simulink model "Simulinkrakata_lusail"  (R2024b)
settings: Solver=VariableStepAuto  StartTime=0.0  StopTime=700  RelTol=1e-3  AbsTol=1e-3
undefined symbols (not defined in the file or in its folder): coast_lookahead, lower_bound, throttle_slew, throttle_val, track_curvature, track_dist, track_slope, upper_bound
libraries: fl_lib x9, nesl_utility x9, sdl_lib x7, simulink x1, ee_lib x1
settings Model: Creator=ACER  LastModifiedBy=ACER
settings SolverCC: AutoScaleAbsTol=off  AlgebraicLoopSolver=TrustRegion  MaxZcPerStep=1
settings DebuggingCC: UnconnectedInputMsg=warning  UnconnectedOutputMsg=warning  UnconnectedLineMsg=warning  SymbolicDimsDataTypeCodeGenerationDiagnostic=none
settings ModelReferenceCC: EnableRefExpFcnMdlSchedulingChecks=on
settings SFSimCC: CustomCodeUndefinedFunction=UseInterfaceOnly
settings RTWCC: GPUComputeCapability=3.5  DLArmComputeVersion=19.05
settings SimscapeCC: SimscapeLogType=all  SimscapeLogSimulationStatistics=on  SimscapeLogDataHistory=10000

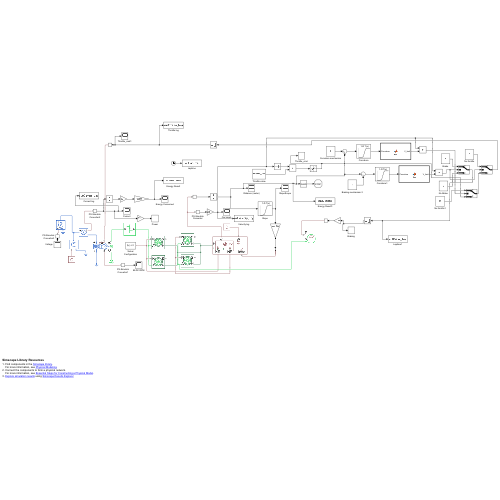
[thumbnail: Simulink's stored preview of the top-level diagram]
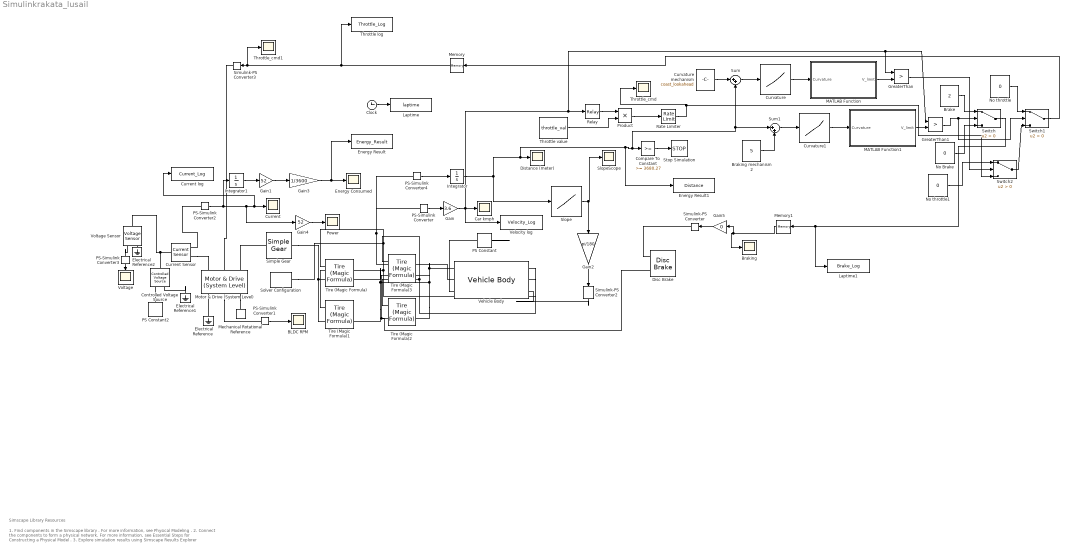
== system Simulinkrakata_lusail ==
  note: 1. Find components in the Simscape library .
      | For more information, see Physical Modeling .
      | 2. Connect the components to form a physical network.
      | For more information, see Essential Steps for Constructing a Physical Model .
      | 3. Explore simulation results using Simscape Results Explorer
  note: Simscape Library Resources
  BLDC RPM : Scope
  Brake : Constant  Value=2
  Braking : Scope
  Braking mechanism 2 : Constant  Value=5
  Car kmph : Scope
  Clock : Clock
  Compare To Constant : simulink/Logic and Bit Operations/Compare To Constant  relop=>=  const=3680.27  OutDataTypeStr=boolean
  Controlled Voltage Source : fl_lib/Electrical/Electrical Sources/Controlled Voltage Source
  Current : Scope
  Current Sensor : fl_lib/Electrical/Electrical Sensors/Current Sensor
  Current log : ToWorkspace  VariableName=Current_Log  SaveFormat=Timeseries  SampleTime=-1
  Curvature : Lookup_n-D  NumberOfTableDimensions=1  BreakpointsForDimension1=track_dist  Table=track_curvature  InternalRulePriority=Speed  RndMeth=Simplest
  Curvature mechanism : Constant  Value=coast_lookahead
  Curvature1 : Lookup_n-D  NumberOfTableDimensions=1  BreakpointsForDimension1=track_dist  Table=track_curvature  InternalRulePriority=Speed  RndMeth=Simplest
  Disc Brake : sdl_lib/Brakes & Detents/Rotational/Disc Brake  r_mean=150 mm  bore=10 mm  n_pads=2  thermal_port=simscape.enum.thermaleffects.omit  mu_static=0.9  mu_coulomb=0.7  temperature_TLU=[280, 300, 320] K  mu_static_TLU=[.9, .8, .7]  mu_coulomb_TLU=[.8, .7, .6]  brkwy_vel=0.1 rad/s  visc_coef=0 N*m*s/rad  thermal_mass=50 kJ/K  temperature_specify=off  temperature_priority=High  temperature=300 K  temperature_nominal_specify=off  temperature_nominal_value=1  temperature_nominal_unit=K
  Distance (meter) : Scope
  Electrical Reference : fl_lib/Electrical/Electrical Elements/Electrical Reference
  Electrical Reference1 : fl_lib/Electrical/Electrical Elements/Electrical Reference
  Electrical Reference2 : fl_lib/Electrical/Electrical Elements/Electrical Reference
  Energy Consumed : Scope
  Energy Result : ToWorkspace  VariableName=Energy_Result  SaveFormat=Timeseries  SampleTime=-1
  Energy Result1 : ToWorkspace  VariableName=Distance  SaveFormat=Timeseries  SampleTime=-1
  Gain : Gain  Gain=3.6
  Gain1 : Gain  Gain=52
  Gain2 : Gain  Gain=pi/180
  Gain3 : Gain  Gain=1/3600
  Gain4 : Gain  Gain=52
  Gain5 : Gain  Gain=0
  GreaterThan : RelationalOperator  Operator=>  OutDataTypeStr=boolean  RndMeth=Simplest  InputSameDT=off
  GreaterThan1 : RelationalOperator  Operator=>  OutDataTypeStr=boolean  RndMeth=Simplest  InputSameDT=off
  Integrator : Integrator
  Integrator1 : Integrator
  Laptime : ToWorkspace  VariableName=laptime  SaveFormat=Timeseries  SampleTime=-1
  Laptime1 : ToWorkspace  VariableName=Brake_Log  SaveFormat=Timeseries  SampleTime=-1
  MATLAB Function : MATLAB Function  TreatAsAtomicUnit=on
  MATLAB Function1 : MATLAB Function  TreatAsAtomicUnit=on
  Mechanical Rotational Reference : fl_lib/Mechanical/Rotational Elements/Mechanical Rotational Reference
  Memory : Memory
  Memory1 : Memory
  Motor & Drive (System Level) : ee_lib/Electromechanical/Motor & Drive (System Level)  torque_speed_param=ee.enum.electromech.envelope.torque_power  overtorque_param=ee.enum.electromech.overtorque.no  T_t=[.09, .08, .07, 0] N*m  T_t_intermittent=[.36, .32, .28, 0] N*m  T_t_2D=[.09, .09, .09; .08, .08, .08; .07, .07, .07; 0, 0, 0] N*m  T_t_intermittent_2D=[.36, .36, .36; .32, .32, .32; .28, .28, .28; 0, 0, 0] N*m  w_t=[0, 3750, 7500, 8000] rpm  vdc_t=[6, 12, 24] V  torque_max=8 N*m  power_max=1000 W  torque_max_intermittent=0.4 N*m  power_max_intermittent=120 W  time_overtorque=30 s  time_recover=60 s  Tc=0.02 s  EnableSwitch=false  losses_param=1  eff=98  w_eff=2500 rpm  T_eff=2 N*m  Piron=0 W  Pbase=0 W  w_eff_vec=[-8000, -4000, 0, 4000, 8000] rpm  T_eff_vec=[0, .03, .06, .09] N*m  v_eff_vec=[100, 250, 400] V  losses_mat=[1.49, 1.67, 2.21, 3.1; .42, .69, 1.14, 2.03; .06, .24, .78, 1.68; .42, .69, 1.14, 2.03; 1.49, 1.67, 2.21, 3.1] W  efficiency_mat=[95, 95, 95, 95; 95, 95, 95, 95; 95, 95, 95, 95; 95, 95, 95, 95; 95, 95, 95, 95]  losses_mat_3D=ones(5, 4, 3) W  efficiency_mat_3D=95 * ones(5, 4, 3)  Res=0 Ohm  J=5e-6 kg*m^2  lam=1e-5 N*m*s/rad  speed0=0 rpm  fault_condition=1  fault_threshold=0.5  faulted_specify=off  faulted_priority=None  faulted=0  faulted_nominal_specify=off  faulted_nominal_value=1  faulted_nominal_unit=1  isSwitchedOff_specify=off  isSwitchedOff_priority=None  isSwitchedOff=0  isSwitchedOff_nominal_specify=off  isSwitchedOff_nominal_value=1  isSwitchedOff_nominal_unit=1  torqueLimitContinuous_specify=off  torqueLimitContinuous_priority=None  torqueLimitContinuous=0 N*m  torqueLimitContinuous_nominal_specify=off  torqueLimitContinuous_nominal_value=1  torqueLimitContinuous_nominal_unit=N*m  alpha=3.93e-3 1/K  Tmeas=25 degC  Tmeas2=125 degC  losses_mat_T2=[1.49, 1.74, 2.49, 3.74; .42, .67, 1.42, 2.67; .06, .31, 1.06, 2.31; .42, .67, 1.42, 2.67; 1.49, 1.74, 2.49, 3.74] W  efficiency_mat_T2=[95, 95, 95, 95; 95, 95, 95, 95; 95, 95, 95, 95; 95, 95, 95, 95; 95, 95, 95, 95]  losses_mat_3D_T2=ones(5, 4, 3) W  efficiency_mat_3D_T2=95 * ones(5, 4, 3)  thermal_mass=100 J/K  initial_temperature=25 degC
  No Brake : Constant  Value=0
  No throttle : Constant  Value=0
  No throttle1 : Constant  Value=0
  PS Constant : fl_lib/Physical Signals/Sources/PS Constant  constant=0 m/s
  PS Constant2 : fl_lib/Physical Signals/Sources/PS Constant  constant=52
  PS-Simulink Converter{,1..4} (5 alike) : nesl_utility/PS-Simulink Converter  PhysicalDomain=network_engine_domain  SubClassName=ps_output  LeftPortType=input  RightPortType=output  PseudoPeriodic=off  Frequencies=[]  VectorFormat=inherit  Unit=inherit  AffineConversion=off
  Power : Scope
  Product : Product
  Rate Limiter : RateLimiter  RisingSlewLimit=throttle_slew  FallingSlewLimit=-10  SampleTimeMode=inherited
  Relay : Relay  OnSwitchValue=upper_bound  OffSwitchValue=lower_bound  OnOutputValue=0  OffOutputValue=1
  Simple Gear : sdl_lib/Gears/Simple Gear  ratio=10  rotation_direction=sdl.enum.shaftOutputDirection.same  friction_model=sdl.enum.gear_efficiencies_load.off  T_noload=0.1 N*m  T_nom=5 N*m  efficiency_nom=0.8  efficiency=0.8  temperature_TLU=[280, 300, 320] K  load_TLU=[1, 5, 10] N*m  efficiency_TLU=[.95, .9, .85]  efficiency_TLU2=[.85, .8, .75; .95, .9, .85; .85, .8, .7]  w_thr=0.01 rad/s  pwr_thr=0.001 W  enable_backlash=false  hardstop_model=simscape.enum.hardstop.smooth  backlash_distance=1e-3 mm  r_base=0.1 m  transition=1e-4 mm  backlash_stiffness=1e6 N/m  backlash_damping=1e3 N*s/m  coeff_rest=0.7  v_tol=0.001 m/s  f_tol=0.001 N  mu_visc=[0, 0] N*m*s/rad  thermal_mass=50 J/K  temperature_specify=off  temperature_priority=High  temperature=300 K  temperature_nominal_specify=off  temperature_nominal_value=1  temperature_nominal_unit=K  x_backlash_specify=off  x_backlash_priority=None  x_backlash=0 mm  x_backlash_nominal_specify=off  x_backlash_nominal_value=1  x_backlash_nominal_unit=mm  f_hardstop_specify=off  f_hardstop_priority=None  f_hardstop=0 N  f_hardstop_nominal_specify=off  f_hardstop_nominal_value=1  f_hardstop_nominal_unit=N  v_backlash_specify=off  v_backlash_priority=None  v_backlash=0 m/s  v_backlash_nominal_specify=off  v_backlash_nominal_value=1  v_backlash_nominal_unit=m/s
  Simulink-PS Converter : nesl_utility/Simulink-PS Converter  PhysicalDomain=network_engine_domain  SubClassName=ps_input  LeftPortType=input  RightPortType=output  PseudoPeriodic=off  Frequencies=[]  NoiseDistribution=none  NoiseParameters=[]  Unit=1  AffineConversion=off  FilteringAndDerivatives=provide  SimscapeFilterOrder=1  InputFilterTimeConstant=0.001  UdotUserProvided=0
  Simulink-PS Converter2 : nesl_utility/Simulink-PS Converter  PhysicalDomain=network_engine_domain  SubClassName=ps_input  LeftPortType=input  RightPortType=output  PseudoPeriodic=off  Frequencies=[]  NoiseDistribution=none  NoiseParameters=[]  Unit=1  AffineConversion=off  FilteringAndDerivatives=provide  SimscapeFilterOrder=1  InputFilterTimeConstant=0.001  UdotUserProvided=0
  Simulink-PS Converter3 : nesl_utility/Simulink-PS Converter  PhysicalDomain=network_engine_domain  SubClassName=ps_input  LeftPortType=input  RightPortType=output  PseudoPeriodic=off  Frequencies=[]  NoiseDistribution=none  NoiseParameters=[]  Unit=1  AffineConversion=off  FilteringAndDerivatives=provide  SimscapeFilterOrder=1  InputFilterTimeConstant=0.001  UdotUserProvided=0
  Slope : Lookup_n-D  NumberOfTableDimensions=1  BreakpointsForDimension1=track_dist  Table=track_slope  InternalRulePriority=Speed  RndMeth=Simplest
  SlopeScope : Scope
  Solver Configuration : nesl_utility/Solver Configuration  PhysicalDomain=network_engine_domain  SubClassName=solver  LeftPortType=input  RightPortType=generic  Tones=[]  Harmonics=[]  SimulateNoise=off  Profile=off  UseLocalSampling=off  EnableSwitchedLinearOptims=on  FrequencyDomain=off  UseCCode=off  RelTol=0.001  AbsTol=1e-06  MinStep=1e-09  ToWorkspace=off  RevertToSquareIcSolve=off  NumHomotopyIterations=100  PhasorMode=off  PhasorModeNumHarmonics=1  ConsistencySolver=NEWTON_XTOL_AFTER_FTOL  IndexReductionMethod=DerivativeReplacement  DoDC=off  ResidualTolerance=1e-09  ConsistencyTolSource=GLOBAL  ConsistencyAbsTol=0.001  ConsistencyRelTol=0.001  ConsistencyTolFactor=0.001  UseLocalSolver=off  LocalSolverChoice=NE_BACKWARD_EULER_ADVANCER  ResolveIndetEquations=on  FunctionEvalNumThread=1  LocalSolverSampleTime=0.001  DoFixedCost=off  MaxNonlinIter=3  MaxModeIter=2  ComputeImpulses=off  ImpulseIterations=2  LinearAlgebra=auto  LinearAlgebraNumThread=0  EquationFormulation=NE_TIME_EF  DelaysMemoryBudget=1024  AutomaticFiltering=on  FilteringTimeConstant=0.001  PartitionStorageMethod=AS_NEEDED  PartitionMemoryBudget=1024  PartitionMethod=ROBUST  MultibodyUseLocalSolver=off  MultibodyLocalSolverChoice=ODE1  MultibodyLocalSolverSampleTime=0.001
  Stop Simulation : Stop
  Sum : Sum  Inputs=|++
  Sum1 : Sum  Inputs=|++
  Switch : Switch  Criteria=u2 > Threshold  SaturateOnIntegerOverflow=off  InputSameDT=off
  Switch1 : Switch  Criteria=u2 > Threshold  SaturateOnIntegerOverflow=off  InputSameDT=off
  Switch2 : Switch  Criteria=u2 > Threshold  SaturateOnIntegerOverflow=off  InputSameDT=off
  Throttle log : ToWorkspace  VariableName=Throttle_Log  SaveFormat=Timeseries  SampleTime=-1
  Throttle value : Constant  Value=throttle_val
  Throttle_cmd : Scope
  Throttle_cmd1 : Scope
  Tire (Magic Formula){,1..3} (4 alike) : sdl_lib/Tires & Vehicles/Tire (Magic Formula)  parameterization=sdl.enum.magic_tire_model.peak  F_z1=3000 N  F_x1=3500 N  kappa1=10  B_m=10  C_m=1.9  D_m=1  E_m=0.97  fz0=4000 N  p_Cx=1.685  p_Dx=[1.21, -.037]  p_Ex=[.344, .095, -.02, 0]  p_Kx=[21.51, -.163, .245]  p_Hx=[-.002, .002]  p_Vx=[0, 0]  rolling_radius_model=sdl.enum.RollingRadiusParameterization.Constant  r_e=0.3 m  r_0=0.3 m  breff=8.39  dreff=0.26  freff=0.074  q_re0=0.99  q_v1=0.008  longvl=17 m/s  cz=5e5 N/m  model_resistance=true  resistance_model=sdl.enum.rollingResistanceParameterization.constant  coeff=0.0015  p_tire=250e3 Pa  alpha=-0.003  beta=0.97  coeff_a=84e-4  coeff_b=6.2e-4 s/m  coeff_c=1.6e-4 s^2/m^2  p_tire0=240e3 Pa  fz0_resistance=4000 N  vH0=16 m/s  q_Sy=[.0082, 0, .0014, .001, 0, 0, 1.08, -.5]  v_thr=0.001 m/s  enable_scaling_coefficients=false  lfzO=1  lcx=1  lmux=1  lex=1  lkx=1  lhx=1  lvx=1  lmy=1  model_compliance=sdl.enum.compliance.off  stiffness=1e6 N/m  damping=1000 N*s/m  model_inertia=sdl.enum.model_inertia.on  inertia=1 kg*m^2  initial_velocity=0 rad/s  vxlow=1 m/s  v_tr_thr=0.1 m/s  kpumin=-1.5  kpumax=1.5
  Vehicle Body : sdl_lib/Tires & Vehicles/Vehicle Body  mass=140 kg  n_w=2  x_f=703 mm  x_r=667 mm  y_c=0.2 m  mass_var=false  g=9.81 m/s^2  liftoff_warning=false  area=0.982 m^2  Cd_var=false  Cd=0.149  rho=1.164 kg/m^3  model_pitch=false  inertia=4000 kg*m^2  suspension_model=sdl.enum.linearTLU.linear  k_f=1e4 N/m  b_f=1e4 N*s/m  k_r=1e4 N/m  b_r=1e4 N*s/m  k_f_TLU=[-2000, -1000, 0, 1000, 2000] N  x_f_TLU=[-.4, -.2, 0, .2, .4] m  b_f_TLU=[-200, -100, 0, 100, 200] N  v_f_TLU=[-4, -2, 0, 2, 4] m/s  k_r_TLU=[-2000, -1000, 0, 1000, 2000] N  x_r_TLU=[-.4, -.2, 0, .2, .4] m  b_r_TLU=[-200, -100, 0, 100, 200] N  v_r_TLU=[-4, -2, 0, 2, 4] m/s  interp_method=simscape.enum.interpolation.linear  extrap_method=simscape.enum.extrapolation.linear  model_hardstop=false  upper_bound_f=.25 m  lower_bound_f=-.25 m  stop_k_f=1e6 N/m  stop_b_f=150 N*s/m  upper_bound_r=.25 m  lower_bound_r=-.25 m  stop_k_r=1e6 N/m  stop_b_r=150 N*s/m  initial_pitch=0 rad  initial_pitch_rate=0 rad/s  v_specify=off  v_priority=High  v=0 m/s  v_nominal_specify=off  v_nominal_value=1  v_nominal_unit=m/s
      settings: InternalSimscapePortConfiguration="{\"Bottom\":[{\"id\":\"NR\",\"label\":\"NR\",\"type\":\"output\"},{\"id\":\"NF\",\"label\":\"NF\",\"type\":\"output\"},{\"id\":\"beta\",\"label\":\"beta\",\"type\":\"input\"}],\"Left\":[{\"id\":\"H\",\"label\":\"H\",\"type\":\"foundation.mechanical.translational.translational\"}],\"Right\":[],\"Top\":[{\"id\":\"V\",\"label\":\"V\",\"type\":\"output\"},{\"id\":\"wind\",\"label\":\"W\",\"type\":\"input\"}]}"
  Velocity log : ToWorkspace  VariableName=Velocity_Log  SaveFormat=Timeseries  SampleTime=-1
  Voltage : Scope
  Voltage Sensor : fl_lib/Electrical/Electrical Sensors/Voltage Sensor
  wires:
  PS-Simulink Converter1/1 -> BLDC RPM/1
  PS-Simulink Converter2/1 -> Integrator1/1, Gain4/1, Current log/1, Current/1
  PS-Simulink Converter3/1 -> Voltage/1
  PS-Simulink Converter4/1 -> Integrator/1
  Integrator/1 -> Slope/1, Energy Result1/1, Sum/2, Sum1/1, Compare To Constant/1, Distance (meter)/1
  PS-Simulink Converter/1 -> Gain/1
  Gain/1 -> Velocity log/1, GreaterThan1/1, GreaterThan/1, Relay/1, Car kmph/1
  Integrator1/1 -> Gain1/1
  Gain1/1 -> Gain3/1
  Slope/1 -> Gain2/1, SlopeScope/1
  Gain2/1 -> Simulink-PS Converter2/1
  Gain3/1 -> Energy Result/1, Energy Consumed/1
  Gain4/1 -> Power/1
  Relay/1 -> Product/1
  Throttle value/1 -> Product/2
  Product/1 -> Rate Limiter/1
  Rate Limiter/1 -> Switch2/3, Throttle_cmd/1
  Compare To Constant/1 -> Stop Simulation/1
  Clock/1 -> Laptime/1
  Curvature mechanism/1 -> Sum/1
  Sum/1 -> Curvature/1
  Curvature/1 -> MATLAB Function/1(Curvature)
  MATLAB Function/1(V_limit) -> GreaterThan/2
  Braking mechanism 2/1 -> Sum1/2
  Sum1/1 -> Curvature1/1
  Curvature1/1 -> MATLAB Function1/1(Curvature)
  MATLAB Function1/1(V_limit) -> GreaterThan1/2
  GreaterThan1/1 -> Switch1/2, Switch/2
  Brake/1 -> Switch/1
  No Brake/1 -> Switch/3
  No throttle/1 -> Switch1/1
  Switch2/1 -> Switch1/3
  GreaterThan/1 -> Switch2/2
  No throttle1/1 -> Switch2/1
  Switch1/1 -> Memory/1
  Switch/1 -> Laptime1/1, Memory1/1
  Memory1/1 -> Gain5/1, Braking/1
  Memory/1 -> Throttle log/1, Throttle_cmd1/1, Simulink-PS Converter3/1
  Gain5/1 -> Simulink-PS Converter/1
  connections:
  Vehicle Body/LConn1 -- Tire (Magic Formula)2/RConn2 -- Tire (Magic Formula)1/RConn2 -- Tire (Magic Formula)/RConn2 -- Tire (Magic Formula)3/RConn2
  Vehicle Body/RConn2 -- Tire (Magic Formula)3/LConn1 -- Tire (Magic Formula)2/LConn1
  Vehicle Body/RConn1 -- Solver Configuration/RConn1 -- Tire (Magic Formula)/LConn1 -- Tire (Magic Formula)1/LConn1
  Tire (Magic Formula)3/LConn2 -- Disc Brake/LConn2 -- Tire (Magic Formula)2/LConn2
  Tire (Magic Formula)/LConn2 -- Tire (Magic Formula)1/LConn2 -- Simple Gear/RConn1
  PS Constant/RConn1 -- Vehicle Body/LConn3
  Vehicle Body/LConn2 -- PS-Simulink Converter4/LConn1 -- PS-Simulink Converter/LConn1
  Motor & Drive (System Level)/RConn3 -- Mechanical Rotational Reference/LConn1
  Electrical Reference/LConn1 -- Motor & Drive (System Level)/RConn1
  Electrical Reference1/LConn1 -- Controlled Voltage Source/RConn2
  Simple Gear/LConn1 -- Motor & Drive (System Level)/LConn3
  Controlled Voltage Source/LConn1 -- Current Sensor/LConn1 -- Voltage Sensor/LConn1
  Current Sensor/RConn2 -- Motor & Drive (System Level)/LConn1
  Current Sensor/RConn1 -- PS-Simulink Converter2/LConn1
  Electrical Reference2/LConn1 -- Voltage Sensor/RConn2
  PS-Simulink Converter3/LConn1 -- Voltage Sensor/RConn1
  Controlled Voltage Source/RConn1 -- PS Constant2/RConn1
  Motor & Drive (System Level)/RConn2 -- PS-Simulink Converter1/LConn1
  Motor & Drive (System Level)/LConn2 -- Simulink-PS Converter3/RConn1
  Simulink-PS Converter2/RConn1 -- Vehicle Body/RConn3
  Simulink-PS Converter/RConn1 -- Disc Brake/LConn1

== matlab function Simulinkrakata_lusail/MATLAB Function1 ==
  data: Curvature input; V_limit output
function V_limit = fcn(Curvature)
    % Parameter Fisika
    mu = 0.8;   % Gesekan ban
    g  = 9.81;  % Gravitasi
    
    % Safety margin (biar gak ngepas banget teorinya)
    margin = 999; 
    
    % Hindari pembagian nol (jalan lurus curvature = 0)
    k = abs(Curvature);
    if k < 0.0001
        k = 0.0001; 
    end
    
    % Rumus Fisika Tikungan
    % V = sqrt(mu * g / k)
    V_limit = sqrt((mu * g) / k) * margin;
    
    % Cap maksimum (misal trek lurus max 120 km/h = 33 m/s)
    if V_limit > 33
        V_limit = 33;
    end
end

== matlab function Simulinkrakata_lusail/MATLAB Function ==
  data: Curvature input; V_limit output
function V_limit = fcn(Curvature)
    % Parameter Fisika
    mu = 0.8;   % Gesekan ban
    g  = 9.81;  % Gravitasi
    
    % Safety margin (biar gak ngepas banget teorinya)
    margin = 999; 
    
    % Hindari pembagian nol (jalan lurus curvature = 0)
    k = abs(Curvature);
    if k < 0.0001
        k = 0.0001; 
    end
    
    % Rumus Fisika Tikungan
    % V = sqrt(mu * g / k)
    V_limit = sqrt((mu * g) / k) * margin;
    
    % Cap maksimum (misal trek lurus max 120 km/h = 33 m/s)
    if V_limit > 33
        V_limit = 33;
    end
end
